simulink model "ps4"  (R2020b)
settings: Solver=VariableStepAuto  StartTime=0.0  StopTime=10.0  RelTol=1e-3
settings Model: Creator=prana  LastModifiedBy=prana

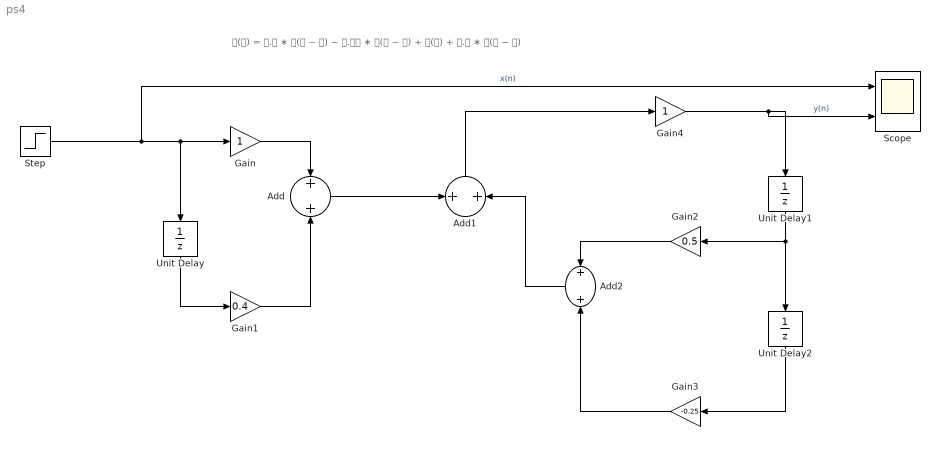
== system ps4 ==
  note: 𝐲(𝐧) = 𝟎.𝟓 ∗ 𝐲(𝐧 − 𝟏) − 𝟎.𝟐𝟓 ∗ 𝐲(𝐧 − 𝟐) + 𝐱(𝐧) + 𝟎.𝟒 ∗ 𝐱(𝐧 − 𝟏)
  Add : Sum
  Add1 : Sum
  Add2 : Sum
  Gain : Gain
  Gain1 : Gain  Gain=0.4
  Gain2 : Gain  Gain=0.5
  Gain3 : Gain  Gain=-0.25
  Gain4 : Gain
  Scope : Scope  NumInputPorts=2
  Step : Step  SampleTime=0
  Unit Delay : UnitDelay  SampleTime=-1  HasFrameUpgradeWarning=on
  Unit Delay1 : UnitDelay  SampleTime=-1  HasFrameUpgradeWarning=on
  Unit Delay2 : UnitDelay  SampleTime=-1  HasFrameUpgradeWarning=on
  wires:
  Step/1 -> Scope/1, Gain/1, Unit Delay/1  "x(n)"
  Unit Delay/1 -> Gain1/1
  Add/1 -> Add1/1
  Add1/1 -> Gain4/1
  Add2/1 -> Add1/2
  Unit Delay1/1 -> Unit Delay2/1, Gain2/1
  Unit Delay2/1 -> Gain3/1
  Gain/1 -> Add/1
  Gain1/1 -> Add/2
  Gain2/1 -> Add2/1
  Gain3/1 -> Add2/2
  Gain4/1 -> Scope/2, Unit Delay1/1  "y(n)"
